simulink model "ros_line_follower_all"  (R2021a)
settings: Solver=FixedStepDiscrete  StartTime=0.0  StopTime=inf  FixedStep=0.05  RelTol=1e-3
model workspace (MAT data in the model file):
  SL_ROS_VariableLengthArrays_MaxSizes.CommonInfo.ArrayTruncateAction = 'EmitWarning'
  SL_ROS_VariableLengthArrays_MaxSizes.MsgTypeMap = containers.Map
  SL_ROS_VariableLengthArrays_MaxSizes.MsgTypeMap.serialization.keys = {'sensor_msgs/Image'}
  SL_ROS_VariableLengthArrays_MaxSizes.MsgTypeMap.serialization.values{1}(1).PropertyName = 'Data'
  SL_ROS_VariableLengthArrays_MaxSizes.MsgTypeMap.serialization.values{1}(1).DataType = 'uint8'
  SL_ROS_VariableLengthArrays_MaxSizes.MsgTypeMap.serialization.values{1}(1).MaxLength = 2764800
  SL_ROS_VariableLengthArrays_MaxSizes.MsgTypeMap.serialization.values{1}(2).PropertyName = 'Encoding'
  SL_ROS_VariableLengthArrays_MaxSizes.MsgTypeMap.serialization.values{1}(2).DataType = 'uint8'
  SL_ROS_VariableLengthArrays_MaxSizes.MsgTypeMap.serialization.values{1}(2).MaxLength = 921600
  SL_ROS_VariableLengthArrays_MaxSizes.MsgTypeMap.serialization.uniformity = 0
  SL_ROS_VariableLengthArrays_MaxSizes.MsgTypeMap.serialization.keyType = 'char'
  SL_ROS_VariableLengthArrays_MaxSizes.MsgTypeMap.serialization.valueType = 'any'
libraries: robotlib x4, visiontextngfix x2, visionconversions x1, deeplib x1, visionsinks x1, pid_lib x1
settings Model: EnablePacing=on  Creator=The MathWorks, Inc.  LastModifiedBy=tkikawad
settings SolverCC: AlgebraicLoopSolver=TrustRegion
settings DataIOCC: ReturnWorkspaceOutputs=off
settings OptimizationCC: LifeSpan=inf  MaxStackSize=64  EfficientTunableParamExpr=on
settings DebuggingCC: ParameterPrecisionLossMsg=none  ParameterTunabilityLossMsg=error  PregeneratedLibrarySubsystemCodeDiagnostic=none  SFExecutionAtInitializationDiag=none  SFMachineParentedDataDiag=warning  ArithmeticOperatorsInVariantConditions=warning
settings HardwareCC: ProdBitPerLong=64  ProdHWDeviceType=Intel->x86-64 (Linux 64)
settings SFSimCC: SimUseLocalCustomCode=off  MATLABDynamicMemAlloc=off  CustomCodeUndefinedFunction=UseInterfaceOnly  SimTargetLang=C++
settings RTWCC: SystemTargetFile=ert.tlc  HardwareBoard=Robot Operating System (ROS)  TLCOptions="-aInlineSetEventsForThisBaseRateFcn=TLC_FALSE -aSuppressMultiTaskScheduler=TLC_FALSE  -aRateBasedStepFcn=0"  TemplateMakefile=ert_default_tmf  GenerateReport=on  RTWUseLocalCustomCode=off  Toolchain=Catkin  IncludeHyperlinkInReport=on  LaunchReport=on  TargetLang=C++  GenerateTraceInfo=on  GenerateTraceReport=on  GenerateTraceReportSl=on  GenerateTraceReportSf=on  GenerateTraceReportEml=on  GenerateWebview=on
settings CodeAppCC: ForceParamTrailComments=on  IgnoreCustomStorageClasses=off  OperatorAnnotations=on  SimulinkDataObjDesc=on  SFDataObjDesc=on  MATLABFcnDesc=on  InsertBlockDesc=on  StateflowObjectComments=on  MATLABSourceComments=on
settings ERTTargetCC: TargetLangStandard=C99 (ISO)  MultiwordLength=2048  SupportVariableSizeSignals=on
settings ConfigComp: CovMetricSettings=dsw  CovSaveCumulativeToWorkspaceVar=on  CovSaveSingleToWorkspaceVar=on  CovExternalEMLEnable=off
settings SimscapeCC: SimscapeNormalizeSystem=off

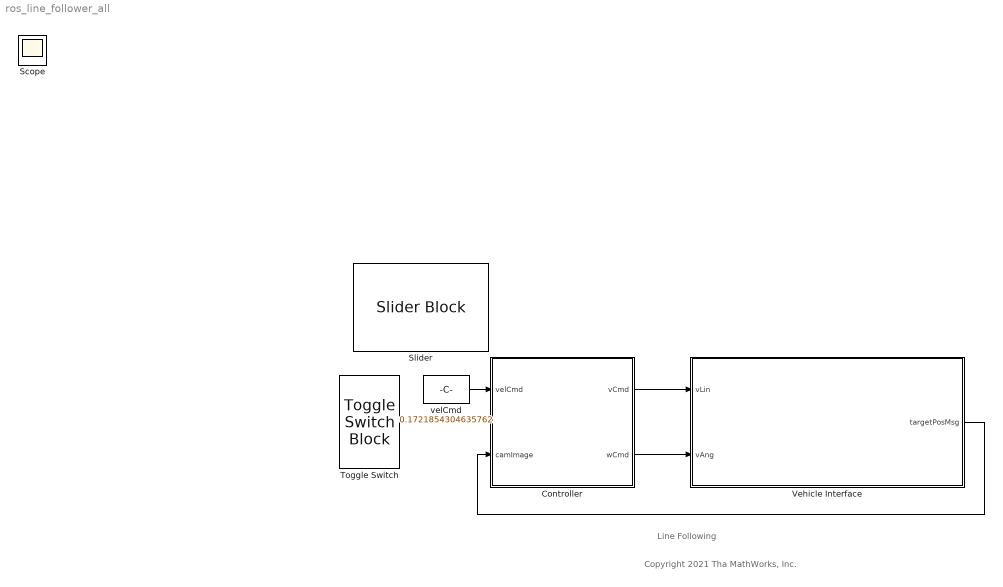
== system ros_line_follower_all ==
  note: Copyright 2021 Tha MathWorks, Inc.
  note: Line Following
  Controller : Subsystem
  Slider : SliderBlock  ScaleMax=1
  Toggle Switch : ToggleSwitchBlock
      settings: Values={{'Off', 'On'}, [0 1]}
  Vehicle Interface : Subsystem
  velCmd : Constant  Value=0.1721854304635762  SampleTime=-1
  Scope : Scope
  wires:
  velCmd/1 -> Controller/1(velCmd)
  Controller/1(vCmd) -> Vehicle Interface/1(vLin)
  Controller/2(wCmd) -> Vehicle Interface/2(vAng)
  Vehicle Interface/1(targetPosMsg) -> Controller/2(camImage)

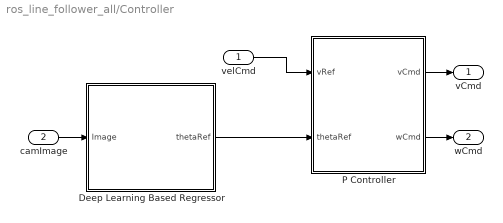
== system ros_line_follower_all/Controller ==
  velCmd : Inport
  camImage : Inport  Port=2
  Deep Learning Based Regressor : Subsystem
  P Controller : Subsystem
  vCmd : Outport
  wCmd : Outport  Port=2
  wires:
  P Controller/2(wCmd) -> wCmd/1
  camImage/1 -> Deep Learning Based Regressor/1(Image)
  velCmd/1 -> P Controller/1(vRef)
  P Controller/1(vCmd) -> vCmd/1
  Deep Learning Based Regressor/1(thetaRef) -> P Controller/2(thetaRef)

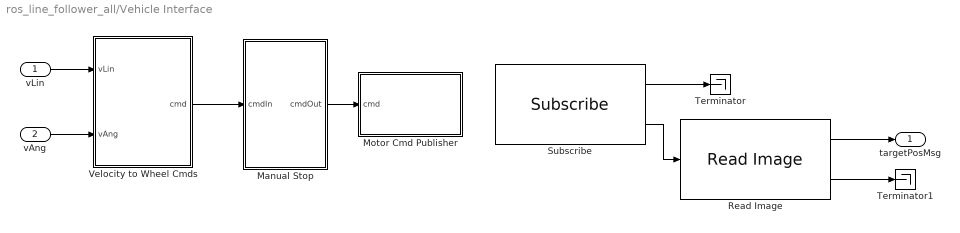
== system ros_line_follower_all/Vehicle Interface ==
  vLin : Inport
  vAng : Inport  Port=2
  Manual Stop : Subsystem
  Motor Cmd Publisher : Subsystem
  Read Image : robotlib/Read Image  MaximumImageSize=[180, 320]  ImageEncoding=bgr8  ShowAlphaOutput=off  ShowErrorCodeOutput=on  VariableSizeOutputs=off
      settings: SourceProductBaseCode=RR
  Subscribe : robotlib/Subscribe  topicSource=Specify your own  topic=/image_raw  messageType=sensor_msgs/Image  SampleTime=-1  legacyBusStruct=off  messageQueueLength=1
  Terminator : Terminator
  Terminator1 : Terminator
  Velocity to Wheel Cmds : MATLAB Function  TreatAsAtomicUnit=on
  targetPosMsg : Outport
  wires:
  vLin/1 -> Velocity to Wheel Cmds/1(vLin)
  Manual Stop/1(cmdOut) -> Motor Cmd Publisher/1(cmd)
  Read Image/1 -> targetPosMsg/1
  Velocity to Wheel Cmds/1(cmd) -> Manual Stop/1(cmdIn)
  Subscribe/1 -> Terminator/1
  vAng/1 -> Velocity to Wheel Cmds/2(vAng)
  Subscribe/2 -> Read Image/1
  Read Image/2 -> Terminator1/1

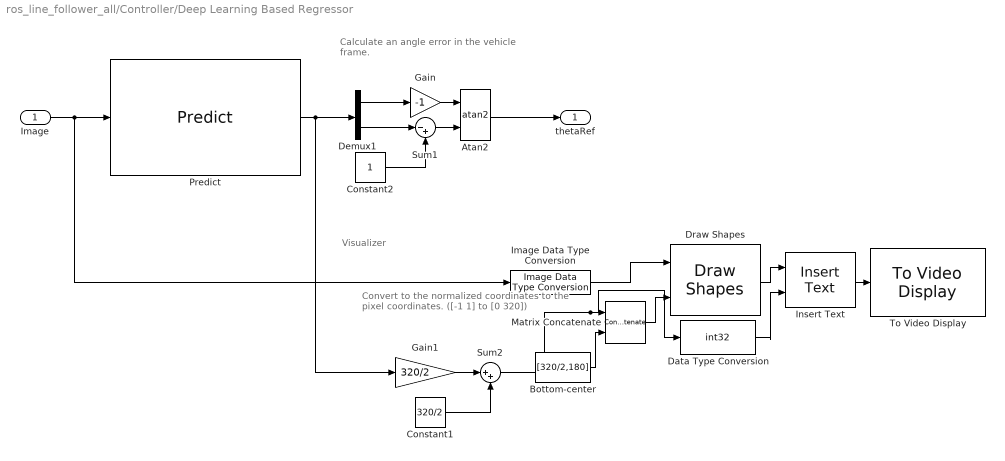
== system ros_line_follower_all/Controller/Deep Learning Based Regressor ==
  note: Visualizer
  note: Calculate an angle error
      | in the vehicle frame.
  note: Convert to the normalized
      | coordinates to
      | the pixel coordinates.
      | ([-1 1] to [0 320])
  Image : Inport
  Atan2 : Trigonometry  Operator=atan2
  Bottom-center : Constant  Value=[320/2,180]  VectorParams1D=off
  Constant1 : Constant  Value=320/2
  Constant2 : Constant  OutDataTypeStr=single
  Data Type Conversion : DataTypeConversion  OutDataTypeStr=int32
  Demux1 : Demux  Outputs=2
  Draw Shapes : visiontextngfix/Draw Shapes  shape=Lines  fill=off  lineWidth=3  fillClrSource=Specify via dialog  display=User-specified value  intensity=200  color=[1,0,0]  opacity=0.6  viewport=Entire image  antialiasing=on  inType=Obsolete  imagePorts=One multidimensional signal  roundingMode=Floor  overflowMode=off  memoryMode=Specify word length  memoryWordLength=16  prodOutputMode=Binary point scaling  prodOutputWordLength=32  prodOutputFracLength=14  memoryFracLength=15
  Gain : Gain  Gain=-1
  Gain1 : Gain  Gain=320/2
  Image Data Type Conversion : visionconversions/Image Data Type Conversion  outDT=single  isSigned=on  wordLen=16  numFracBits=0
      settings: SourceProductBaseCode=VP
  Insert Text : visiontextngfix/Insert Text  inputType=Obsolete  theText="'  Predicted point'"  getTextLocFrom=Input port  textLoc=[1 1]  getTextColorFrom=Specify via dialog  textColor=[1,0,0]  getTextIntensityFrom=Specify via dialog  textIntensity=0  getTextOpacityFrom=Specify via dialog  textOpacity=1.0  dummyVar2=0  dummyVar3=0  dummyVar4=0  imagePorts=One multidimensional signal  isInputTransposed=off  fontFace=LucidaSansRegular  dummyVar1=0  blockFontSize=12  antiAliased=on
      settings: SourceProductBaseCode=VP
  Matrix Concatenate : Concatenate  Mode=Multidimensional array  ConcatenateDimension=2
  Predict : deeplib/Predict  Network=Network from MAT-file  NetworkFunction=squeezenet  NetworkFilePath=mynet_new.mat  MiniBatchSize=1  InputDataFormats={ '', '' }  Predictions=on  Activations={}  ForceInterpretedSim=off  EnableDLNetwork=off
      settings: SourceProductBaseCode=NN
  Sum1 : Sum  Inputs=|-+
  Sum2 : Sum  Inputs=|++
  To Video Display : visionsinks/To Video Display  windowSizeMode=Normal  openAtMdlStart=on  fullScreen=off  videoWindowX=-764  videoWindowY=513  saveWindowSize=off  videoWindowWidth=320  videoWindowHeight=180  inputColorFormat=RGB  inputType=Obsolete  imagePorts=One multidimensional signal  OutputDevice=On-screen video monitor  dataOrg=Column-major  isWindowOpen=off
  thetaRef : Outport
  wires:
  Demux1/1 -> Gain/1
  Atan2/1 -> thetaRef/1
  Demux1/2 -> Sum1/1
  Sum1/1 -> Atan2/2
  Constant2/1 -> Sum1/2
  Gain1/1 -> Sum2/1
  Sum2/1 -> Data Type Conversion/1, Matrix Concatenate/1
  Constant1/1 -> Sum2/2
  Predict/1 -> Gain1/1, Demux1/1
  Image/1 -> Predict/1, Image Data Type Conversion/1
  Draw Shapes/1 -> Insert Text/1
  Image Data Type Conversion/1 -> Draw Shapes/1
  Matrix Concatenate/1 -> Draw Shapes/2
  Bottom-center/1 -> Matrix Concatenate/2
  Insert Text/1 -> To Video Display/1
  Data Type Conversion/1 -> Insert Text/2
  Gain/1 -> Atan2/1

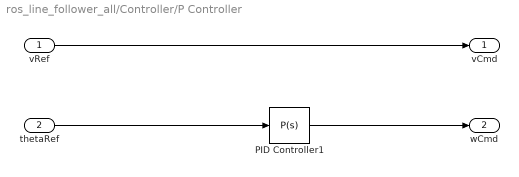
== system ros_line_follower_all/Controller/P Controller ==
  vRef : Inport
  thetaRef : Inport  Port=2
  PID Controller1 : pid_lib/PID Controller  Controller=P  Form=Parallel  TimeDomain=Continuous-time  UseExternalTs=off  SampleTime=0.01  IntegratorMethod=Forward Euler  FilterMethod=Forward Euler  ControllerParametersSource=internal  P=2  I=0.01  D=0.5  UseFilter=on  N=100  TunerSelectOption=Transfer Function Based (PID Tuner App)  InitialConditionSource=internal  InitialConditionForIntegrator=0  InitialConditionForFilter=0  DifferentiatorICPrevScaledInput=0  ExternalReset=none  TrackingMode=off  Kt=1  LimitOutput=off  SatLimitsSource=internal  UpperSaturationLimit=inf  LowerSaturationLimit=-inf  LinearizeAsGain=on  AntiWindupMode=none  Kb=1  POutMin=[]  POutMax=[]  IOutMin=[]  IOutMax=[]  DOutMin=[]  DOutMax=[]  NOutMin=[]  NOutMax=[]  SumOutMin=[]  SumOutMax=[]  SaturationOutMin=[]  SaturationOutMax=[]  PParamMin=[]  PParamMax=[]  IParamMin=[]  IParamMax=[]  DParamMin=[]  DParamMax=[]  NParamMin=[]  NParamMax=[]  KbParamMin=[]  KbParamMax=[]  KtParamMin=[]  KtParamMax=[]  KbOutMin=[]  KbOutMax=[]  KtOutMin=[]  KtOutMax=[]  IntegratorOutMin=[]  IntegratorOutMax=[]  FilterOutMin=[]  FilterOutMax=[]  SumI1OutMin=[]  SumI1OutMax=[]  SumI2OutMin=[]  SumI2OutMax=[]  SumI3OutMin=[]  SumI3OutMax=[]  SumI4OutMin=[]  SumI4OutMax=[]  SumDOutMin=[]  SumDOutMax=[]  DifferentiatorOutMin=[]  DifferentiatorOutMax=[]  FilterDiffOutCoefMin=[]  FilterDiffOutCoefMax=[]  ReciprocalOutMin=[]  ReciprocalOutMax=[]  SumDenOutMin=[]  SumDenOutMax=[]  SumNumOutMin=[]  SumNumOutMax=[]  DivideOutMin=[]  DivideOutMax=[]  UdiffTsProdOutMin=[]  UdiffTsProdOutMax=[]  NTsProdOutMin=[]  NTsProdOutMax=[]  UintegralTsProdOutMin=[]  UintegralTsProdOutMax=[]  UngainTsProdOutMin=[]  UngainTsProdOutMax=[]  IntegratorContinuousStateAttributes=''  IntegratorStateMustResolveToSignalObject=off  IntegratorRTWStateStorageClass=Auto  FilterContinuousStateAttributes=''  FilterStateMustResolveToSignalObject=off  FilterRTWStateStorageClass=Auto  ParallelPVariant=InternalParameters  IdealPVariant=Disabled  IVariant=Disabled  DVariant=Disabled  IntegratorVariant=Disabled  SatVariant=Disabled  AWVariant=Disabled  PCopyVariant=Disabled  TRVariant=Disabled  FdbkBlocksVariant=Forward  IdealPFdbkVariant=Disabled  SatFdbkVariant=Disabled  DerivativeFilterVariant=Disabled  NVariant=Disabled  NCopyVariant=Disabled_SignalSpec  FilterICVariant=Disabled  IntegratorICVariant=Disabled  ExternalResetVariant=Disabled  TRSumVariant=Passthrough  SumFdbkVariant=Disabled  SumVariant=Passthrough_P  TsampFilterVariant=InternalTs  TsampNgainVariant=Passthrough  TsampIntegralVariant=Disabled_SignalSpec  ExternalSaturationOutDataTypeStr=Inherit: Same as second input
  vCmd : Outport
  wCmd : Outport  Port=2
  wires:
  vRef/1 -> vCmd/1
  PID Controller1/1 -> wCmd/1
  thetaRef/1 -> PID Controller1/1

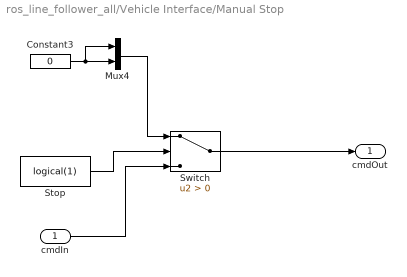
== system ros_line_follower_all/Vehicle Interface/Manual Stop ==
  cmdIn : Inport
  Constant3 : Constant  Value=0  OutDataTypeStr=single  SampleTime=-1
  Mux4 : Mux  Inputs=2
  Stop : Constant  Value=logical(1)  SampleTime=-1
  Switch : Switch  Criteria=u2 > Threshold
  cmdOut : Outport
  wires:
  Mux4/1 -> Switch/1
  Constant3/1 -> Mux4/1, Mux4/2
  cmdIn/1 -> Switch/3
  Stop/1 -> Switch/2
  Switch/1 -> cmdOut/1

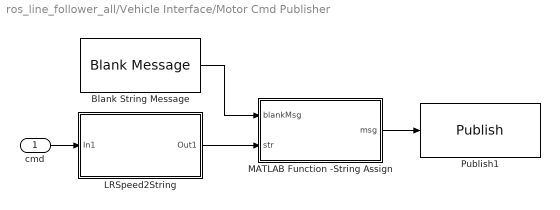
== system ros_line_follower_all/Vehicle Interface/Motor Cmd Publisher ==
  cmd : Inport
  Blank String Message : robotlib/Blank Message  messageClass=Message  entityType=std_msgs/String  messageType=std_msgs/String  SampleTime=inf  legacyBusStruct=off
  LRSpeed2String : Subsystem
  MATLAB Function -String Assign : MATLAB Function  TreatAsAtomicUnit=on
  Publish1 : robotlib/Publish  topicSource=Specify your own  topic=/jetbot_motors/cmd_raw  messageType=std_msgs/String  legacyBusStruct=off  messageQueueLength=1
  wires:
  MATLAB Function -String Assign/1(msg) -> Publish1/1
  Blank String Message/1 -> MATLAB Function -String Assign/1(blankMsg)
  LRSpeed2String/1(Out1) -> MATLAB Function -String Assign/2(str)
  cmd/1 -> LRSpeed2String/1(In1)

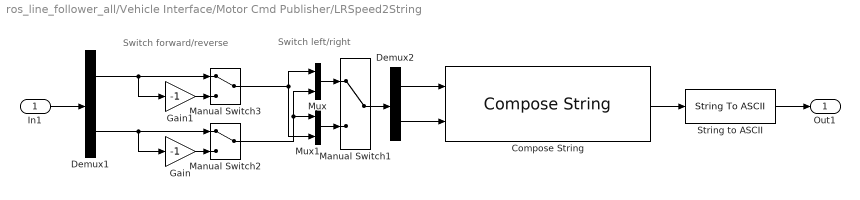
== system ros_line_follower_all/Vehicle Interface/Motor Cmd Publisher/LRSpeed2String ==
  note: Switch left/right
  note: Switch forward/reverse
  In1 : Inport
  Compose String : ComposeString  Format="\"speed[ %+1.4f,%+1.4f ]\""
  Demux1 : Demux  Outputs=2
  Demux2 : Demux  Outputs=2
  Gain : Gain  Gain=-1
  Gain1 : Gain  Gain=-1
  Manual Switch1 : ManualSwitch
  Manual Switch2 : ManualSwitch
  Manual Switch3 : ManualSwitch
  Mux : Mux  Inputs=2
  Mux1 : Mux  Inputs=2
  String to ASCII : StringToASCII
  Out1 : Outport  VectorParamsAs1DForOutWhenUnconnected=off
  wires:
  Demux2/1 -> Compose String/1
  Demux2/2 -> Compose String/2
  In1/1 -> Demux1/1
  Compose String/1 -> String to ASCII/1
  String to ASCII/1 -> Out1/1
  Demux1/2 -> Gain/1, Manual Switch2/1
  Gain/1 -> Manual Switch2/2
  Gain1/1 -> Manual Switch3/2
  Demux1/1 -> Gain1/1, Manual Switch3/1
  Manual Switch1/1 -> Demux2/1
  Mux/1 -> Manual Switch1/1
  Mux1/1 -> Manual Switch1/2
  Manual Switch3/1 -> Mux/1, Mux1/2
  Manual Switch2/1 -> Mux/2, Mux1/1

== matlab function ros_line_follower_all/Vehicle Interface/Velocity to Wheel Cmds ==
  data: vLin input; cmd output; vAng input
function cmd = vel2wheel(vLin,vAng)
%#codegen
d = 0.05125*2;
r = 0.03;

if abs(vAng) > 2
    vl = -d*vAng/2;
    vr =  d*vAng/2;
else
    vl = vLin - d*vAng/2;
    vr = vLin + d*vAng/2;
end
wl = vl / r;
wr = vr / r;
wlCmd = funcl(wl);
wrCmd = funcr(wr);
cmd = [wlCmd,wrCmd];

    function wCmd = funcl(w)
        wCmd = min(max(w*0.1,-1),1);
    end
    function wCmd = funcr(w)
        wCmd = min(max(w*0.096,-1),1);
    end
end

== matlab function ros_line_follower_all/Vehicle Interface/Motor Cmd Publisher/MATLAB Function -String Assign ==
  data: blankMsg input; msg output Bus: SL_Bus_ros_line_follower_all_std_msgs_String; str input
function msg = assignStringInput(blankMsg, str)
% assignStringInput - Assign a string in a ROS message to specified input string
%
% MSG = assignStringInput(blankMsg, STR) assigns the input string, STR, to
%  a string field in the ROS message, blankMsg, and outputs the updated
%  ROS message.
%
%  Inputs
%    blankMsg: A bus for a 'std_msgs/String' message. This is 
%        used to initialize the output.
%    str: An array of uint8 that will be assigned to the 'Data' field
%        in blankMsg. The entire array is assumed to be a valid sequence of
%        character ASCII values.
% 
%  Outputs:
%    msg: A bus for a 'std_msgs/String' message, with the 'Data'
%        field set to a string.

%   Copyright 2015 The MathWorks, Inc.
%#codegen

% Note: The datatype of 'msg' has been explicitly set to the appropriate 
% Simulink bus type ("Bus: SL_Bus_robotROSMessageUsageExample_std_msgs_String"). 
%
% If the model name is changed, the datatype needs to be changed as well:
%   1) Click "Edit Data" in the Editor toolstrip to open "Ports and Data Manager"
%   2) Select "msg". From the "Type" dropdown, select "--- Refresh data types ---"
%   3) Set datatype to "Bus: SL_Bus_<modelname>_std_msgs_String"
    
msg = blankMsg;

% msg (std_msgs/String) consists of
%           Data : array of type uint8
%   Data_SL_Info : struct with fields CurrentLength, ReceivedLength
strLength = length(str);
msg.Data(1:strLength) = uint8(str);
msg.Data_SL_Info.CurrentLength = uint32(strLength);
